simulink model "SampHold"  (R2022b)
settings: Solver=ode45  StartTime=0.0  StopTime=9999.0  MaxStep=.005  RelTol=1e-6  AbsTol=1e-6
settings Model: Creator=vise  LastModifiedBy=rxw14
settings SolverCC: AutoScaleAbsTol=off  InitialStep=.0001  AlgebraicLoopSolver=TrustRegion
settings DataIOCC: SaveFormat=Array  SignalLoggingSaveFormat=ModelDataLogs  ReturnWorkspaceOutputs=off
settings OptimizationCC: BooleanDataType=off  ExpressionDepthLimit=2147483647  InitFltsAndDblsToZero=on  LifeSpan=inf
settings DebuggingCC: SaveWithParameterizedLinksMsg=none  UnderspecifiedInitializationDetection=Classic  MergeDetectMultiDrivingBlocksExec=none  SignalResolutionControl=TryResolveAllWithWarning  MultiTaskDSMMsg=warning  MultiTaskCondExecSysMsg=none  FcnCallInpInsideContextMsg=warning  UnconnectedInputMsg=warning  UnconnectedOutputMsg=warning  UnconnectedLineMsg=warning  StateNameClashWarn=warning  SFUnexpectedBacktrackingDiag=warning  SFNoUnconditionalDefaultTransitionDiag=warning  SFExecutionAtInitializationDiag=none  SFMachineParentedDataDiag=warning  ArithmeticOperatorsInVariantConditions=warning
settings HardwareCC: ProdBitPerPointer=32  ProdBitPerSizeT=32  ProdBitPerPtrDiffT=32  ProdLargestAtomicFloat=None  ProdIntDivRoundTo=Undefined  ProdEndianess=Unspecified  ProdWordSize=32  ProdHWDeviceType=32-bit Generic  TargetUnknown=on
settings ModelReferenceCC: EnableRefExpFcnMdlSchedulingChecks=on  PropagateSignalLabelsOutOfModel=off
settings SFSimCC: SimUseLocalCustomCode=off  CustomCodeUndefinedFunction=UseInterfaceOnly
settings RTWCC: TemplateMakefile=grt_unix.tmf  RTWUseLocalCustomCode=off
settings CodeAppCC: StateflowObjectComments=on
settings GRTTargetCC: TargetLangStandard=C89/C90 (ANSI)  CombineOutputUpdateFcns=off  GRTInterface=on
settings ConfigComp: CovMetricSettings=dw  CovSaveCumulativeToWorkspaceVar=on  CovSaveSingleToWorkspaceVar=on  CovExternalEMLEnable=off

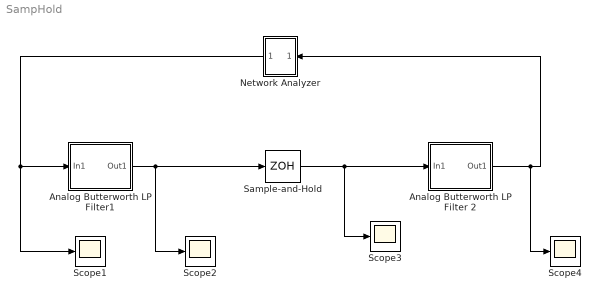
== system SampHold ==
  Analog Butterworth LP Filter 2 : Subsystem  mask(buttap){MaskParam1=0.45*2*pi, MaskParam2=20}
      mask prompts: MaskParam1 "Cutoff frequency (rad/sec)"; MaskParam2 "Order"
      mask help:
      | Analog Butterworth low pass filter.
      |
      | (Requires Signal Processing Toolbox)
      mask init:
      | [z,p,k]=buttap(MaskParam2); z=MaskParam1*z; p=MaskParam1*p; k=real(prod(-p)); [num,den]=zp2tf(z,p,k); w=logspace(log10(MaskParam1/10),log10(10*MaskParam1),20); h=freqs(num,den,w);
      mask Help: Butterworth low pass filter using MATLAB's butter command.
      mask Display: plot(20*log10(w),20*log10(abs(h)))
  Analog Butterworth LP Filter1 : Subsystem  mask(buttap){MaskParam1=0.45*2*pi, MaskParam2=20}
      mask prompts: MaskParam1 "Cutoff frequency (rad/sec)"; MaskParam2 "Order"
      mask help:
      | Analog Butterworth low pass filter.
      |
      | (Requires Signal Processing Toolbox)
      mask init:
      | [z,p,k]=buttap(MaskParam2); z=MaskParam1*z; p=MaskParam1*p; k=real(prod(-p)); [num,den]=zp2tf(z,p,k); w=logspace(log10(MaskParam1/10),log10(10*MaskParam1),20); h=freqs(num,den,w);
      mask Help: Butterworth low pass filter using MATLAB's butter command.
      mask Display: plot(20*log10(w),20*log10(abs(h)))
  Network Analyzer : Subsystem  mask(Network Analyzer){MaskParam1=512, MaskParam2=0.1}
      mask prompts: MaskParam1 "Number of sample points:"; MaskParam2 "Sampling period (sec):"
      mask init:
      | max_freq=0.9*pi/MaskParam2;N=MaskParam1;T_s=MaskParam2;const=2*pi/(MaskParam1*MaskParam2);window1=0.5*MaskParam1*MaskParam2;window2=MaskParam1*MaskParam2;
      mask Help: Estimates frequency response of system using chirp input. Used for EE438. See Prof. Bouman.
      mask Display: plot(0,0,100,100,[11,93,93,11,11],[90,90,40,40,90],[80,60,40,20],[50,79,50,80])
  Sample-and-Hold : ZeroOrderHold
  Scope{1..4} (4 alike) : Scope
  wires:
  Analog Butterworth LP Filter 2/1(Out1) -> Scope4/1, Network Analyzer/1(Inport)
  Network Analyzer/1(Outport) -> Scope1/1, Analog Butterworth LP Filter1/1(In1)
  Analog Butterworth LP Filter1/1(Out1) -> Scope2/1, Sample-and-Hold/1
  Sample-and-Hold/1 -> Scope3/1, Analog Butterworth LP Filter 2/1(In1)

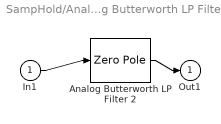
== system SampHold/Analog Butterworth LP Filter 2 ==
  In1 : Inport
  Analog Butterworth LP Filter 2 : ZeroPole  Zeros=z  Poles=p  Gain=k
  Out1 : Outport
  wires:
  In1/1 -> Analog Butterworth LP Filter 2/1
  Analog Butterworth LP Filter 2/1 -> Out1/1

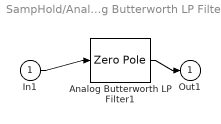
== system SampHold/Analog Butterworth LP Filter1 ==
  In1 : Inport
  Analog Butterworth LP Filter1 : ZeroPole  Zeros=z  Poles=p  Gain=k
  Out1 : Outport
  wires:
  In1/1 -> Analog Butterworth LP Filter1/1
  Analog Butterworth LP Filter1/1 -> Out1/1

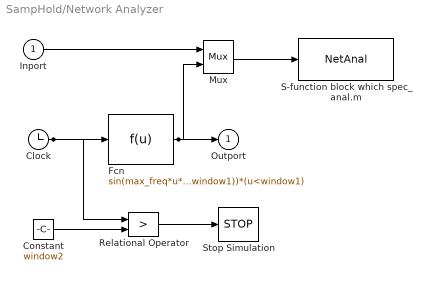
== system SampHold/Network Analyzer ==
  Inport : Inport
  Clock : Clock
  Constant : Constant  Value=window2
  Fcn : Fcn  Expr=sin(max_freq*u*u/(2*window1))*(0.54+0.46*cos(pi*u/window1))*(u<window1)
  Mux : Mux  Inputs=2
  Relational Operator : RelationalOperator  Operator=>
  S-function block which spec_anal.m : S-Function  FunctionName=NetAnal  Parameters=N,T_s  SFunctionDeploymentMode=off  EnableBusSupport=off
  Stop Simulation : Stop
  Outport : Outport  InitialOutput=0
  wires:
  Relational Operator/1 -> Stop Simulation/1
  Clock/1 -> Relational Operator/1, Fcn/1
  Constant/1 -> Relational Operator/2
  Fcn/1 -> Outport/1, Mux/2
  Mux/1 -> S-function block which spec_anal.m/1
  Inport/1 -> Mux/1
